simulink model "Prj1CDig"  (R2026a)
settings: Solver=ode45  StopTime=3000  RelTol=1e-6  EnableMultiTasking=on
values from neighbouring files (symbols this model uses):
  A = (Tz-Tp1)/(Tp2-Tp1)    (= 0.341133511235)    [Prj1CDig_m.m]    (also in sim_params_Prj1CDig.m = (modelo.Tz - modelo.Tp1)/(modelo.Tp2 - modelo.Tp1))
  B = 1 - A    (= 0.658866488765)    [Prj1CDig_m.m]    (also in sim_params_Prj1CDig.m = 1 - A)
  I = -(P*Z-P)/Tc    (= 0.0311935506201)    [Prj1CDig_m.m]    (also in sim_params_Prj1CDig.m = 3.2801)
  modelo = procest(data, modelo_init)    [AnaliseCDig.m]
  P = 0.909    [Prj1CDig_m.m]    (also in sim_params_Prj1CDig.m = -0.101909525131)
  PO = 60    [Prj1CDig_m.m]    (also in sim_params_Prj1CDig.m)
  Ta = 27    [Prj1CDig_m.m]    (also in sim_params_Prj1CDig.m = 23)
  Ts = 1    [AnaliseCDig.m]    (also in Prj1CDig_m.m)
  w0 = 0.09817477042468    (= 0.0981747704247)    [Prj1CDig_m.m]    (also in sim_params_Prj1CDig.m = 0.098)
settings Model: Creator=Adolfo  LastModifiedBy=jhdel
settings SolverCC: ZeroCrossControl=DisableAll
settings DataIOCC: MaxDataPoints=25000  SignalLoggingSaveFormat=ModelDataLogs
settings OptimizationCC: BooleanDataType=off  InitFltsAndDblsToZero=on
settings DebuggingCC: SaveWithParameterizedLinksMsg=none  UnderspecifiedInitializationDetection=Classic  SignalResolutionControl=TryResolveAllWithWarning  MultiTaskDSMMsg=warning  MultiTaskCondExecSysMsg=none
settings HardwareCC: ProdHWDeviceType=32-bit Generic  TargetUnknown=on
settings GRTTargetCC: TargetFcnLib=ansi_tfl_tmw.mat  CombineOutputUpdateFcns=off  GRTInterface=on

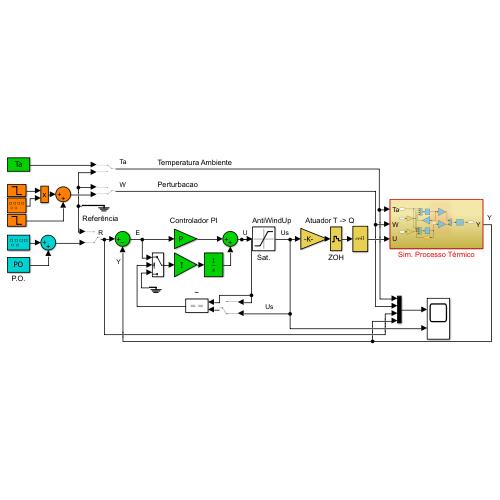
[thumbnail: Simulink's stored preview of the top-level diagram]
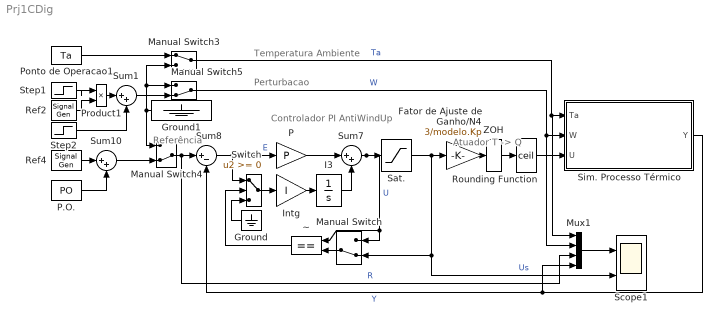
== system Prj1CDig ==
  note: Temperatura Ambiente
  note: Atuador T -> Q
  note: Referência
  note: Controlador PI AntiWindUp
  note: Perturbacao
  Fator de Ajuste de Ganho/N4 : Gain  Gain=3/modelo.Kp  SaturateOnIntegerOverflow=on  OutDataTypeStr=Inherit: Same as input  ParamDataTypeStr=Inherit: Same as input
  Ground : Ground
  Ground1 : Ground
  I3 : Integrator
  Intg : Gain  Gain=I
  Manual Switch : ManualSwitch  CurrentSetting=0
  Manual Switch3 : ManualSwitch
  Manual Switch4 : ManualSwitch  CurrentSetting=0
  Manual Switch5 : ManualSwitch  CurrentSetting=0
  Mux1 : Mux
  P : Gain  Gain=P
  P.O. : Constant  Value=PO
  Ponto de Operacao1 : Constant  Value=Ta
  Product1 : Product  RndMeth=Zero
  Ref2 : SignalGenerator  Frequency=w0  Units=rad/sec
  Ref4 : SignalGenerator  WaveForm=square  Amplitude=5  Frequency=.00125
  Rounding Function : Rounding  Operator=ceil
  Sat. : Saturate  UpperLimit=12  LowerLimit=0
  Scope1 : Scope  NumInputPorts=2
      settings: TimeSpan=3000  ActiveDisplayYMinimum=-18.75  ActiveDisplayYMaximum=68.75  DataLoggingMaxPoints=30000
  Sim. Processo Térmico : Subsystem
  Step1 : Step  Time=2200  FinalValue=-5  SampleTime=0
  Step2 : Step  Time=1100  FinalValue=-5  SampleTime=0
  Sum1 : Sum  Inputs=|++
  Sum10 : Sum  Inputs=|++
  Sum7 : Sum  Inputs=|++
  Sum8 : Sum  Inputs=|+-
  Switch : Switch  SaturateOnIntegerOverflow=off  InputSameDT=off
  ZOH : ZeroOrderHold  SampleTime=Ts
  ~ : RelationalOperator  Operator===  OutDataTypeStr=boolean  InputSameDT=off
  wires:
  Sat./1 -> Manual Switch/2, Scope1/2, Fator de Ajuste de Ganho/N4/1  "Us"
  P.O./1 -> Sum10/2
  Sum7/1 -> ~/1, Manual Switch/1, Sat./1  "U"
  Ref4/1 -> Sum10/1
  ZOH/1 -> Rounding Function/1
  Intg/1 -> I3/1
  Switch/1 -> Intg/1
  P/1 -> Sum7/1
  Ground/1 -> Switch/3
  I3/1 -> Sum7/2
  Sum8/1 -> Switch/1, P/1  "E"
  Rounding Function/1 -> Sim. Processo Térmico/3(U)
  Fator de Ajuste de Ganho/N4/1 -> ZOH/1
  ~/1 -> Switch/2
  Manual Switch5/1 -> Mux1/2, Sim. Processo Térmico/2(W)  "W"
  Manual Switch/1 -> ~/2
  Sim. Processo Térmico/1(Y) -> Mux1/4, Sum8/2  "Y"
  Manual Switch3/1 -> Mux1/1, Sim. Processo Térmico/1(Ta)  "Ta"
  Ground1/1 -> Manual Switch3/2, Manual Switch5/1, Manual Switch4/1
  Manual Switch4/1 -> Mux1/3, Sum8/1  "R"
  Step1/1 -> Product1/1
  Ref2/1 -> Product1/2
  Sum1/1 -> Manual Switch5/2
  Ponto de Operacao1/1 -> Manual Switch3/1
  Sum10/1 -> Manual Switch4/2
  Mux1/1 -> Scope1/1
  Step2/1 -> Sum1/2
  Product1/1 -> Sum1/1

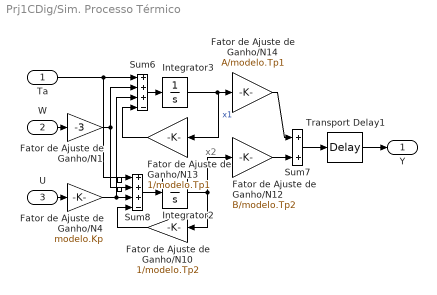
== system Prj1CDig/Sim. Processo Térmico ==
  note: x2
  Ta : Inport
  W : Inport  Port=2
  U : Inport  Port=3
  Fator de Ajuste de Ganho/N1 : Gain  Gain=-3  SaturateOnIntegerOverflow=on  OutDataTypeStr=Inherit: Same as input  ParamDataTypeStr=Inherit: Same as input
  Fator de Ajuste de Ganho/N10 : Gain  Gain=1/modelo.Tp2  SaturateOnIntegerOverflow=on  OutDataTypeStr=Inherit: Same as input  ParamDataTypeStr=Inherit: Same as input
  Fator de Ajuste de Ganho/N12 : Gain  Gain=B/modelo.Tp2  SaturateOnIntegerOverflow=on  OutDataTypeStr=Inherit: Same as input  ParamDataTypeStr=Inherit: Same as input
  Fator de Ajuste de Ganho/N13 : Gain  Gain=1/modelo.Tp1  SaturateOnIntegerOverflow=on  OutDataTypeStr=Inherit: Same as input  ParamDataTypeStr=Inherit: Same as input
  Fator de Ajuste de Ganho/N14 : Gain  Gain=A/modelo.Tp1  SaturateOnIntegerOverflow=on  OutDataTypeStr=Inherit: Same as input  ParamDataTypeStr=Inherit: Same as input
  Fator de Ajuste de Ganho/N4 : Gain  Gain=modelo.Kp  SaturateOnIntegerOverflow=on  OutDataTypeStr=Inherit: Same as input  ParamDataTypeStr=Inherit: Same as input
  Integrator2 : Integrator  InitialCondition=Ta*modelo.Tp2
  Integrator3 : Integrator  InitialCondition=Ta*modelo.Tp1
  Sum6 : Sum  Inputs=+++-
  Sum7 : Sum  InputSameDT=on  SaturateOnIntegerOverflow=on  OutDataTypeStr=Inherit: Same as first input
  Sum8 : Sum  Inputs=+++-
  Transport Delay1 : TransportDelay  DelayTime=modelo.Td  InitialOutput=Ta  PadeOrder=2
  Y : Outport
  wires:
  Sum7/1 -> Transport Delay1/1
  Fator de Ajuste de Ganho/N12/1 -> Sum7/2
  Fator de Ajuste de Ganho/N13/1 -> Sum6/4
  Sum8/1 -> Integrator2/1
  Sum6/1 -> Integrator3/1
  Fator de Ajuste de Ganho/N10/1 -> Sum8/4
  U/1 -> Fator de Ajuste de Ganho/N4/1
  Fator de Ajuste de Ganho/N14/1 -> Sum7/1
  Integrator3/1 -> Fator de Ajuste de Ganho/N14/1, Fator de Ajuste de Ganho/N13/1  "x1"
  Integrator2/1 -> Fator de Ajuste de Ganho/N12/1, Fator de Ajuste de Ganho/N10/1
  Ta/1 -> Sum6/1, Sum8/1
  W/1 -> Fator de Ajuste de Ganho/N1/1
  Fator de Ajuste de Ganho/N4/1 -> Sum8/3, Sum6/3
  Transport Delay1/1 -> Y/1
  Fator de Ajuste de Ganho/N1/1 -> Sum6/2, Sum8/2
